simulink model "deep_sim_0"  (R2025b)
settings: Solver=FixedStepAuto  StartTime=0.0  StopTime=300  FixedStep=.01  RelTol=1e-3
undefined symbols (not defined in the file or in its folder): battery_builder_rtmsupport, gcbh
libraries: Batteries_lib x15, nesl_utility x5, fl_lib x4, ee_lib x1
(part 2 of 2)

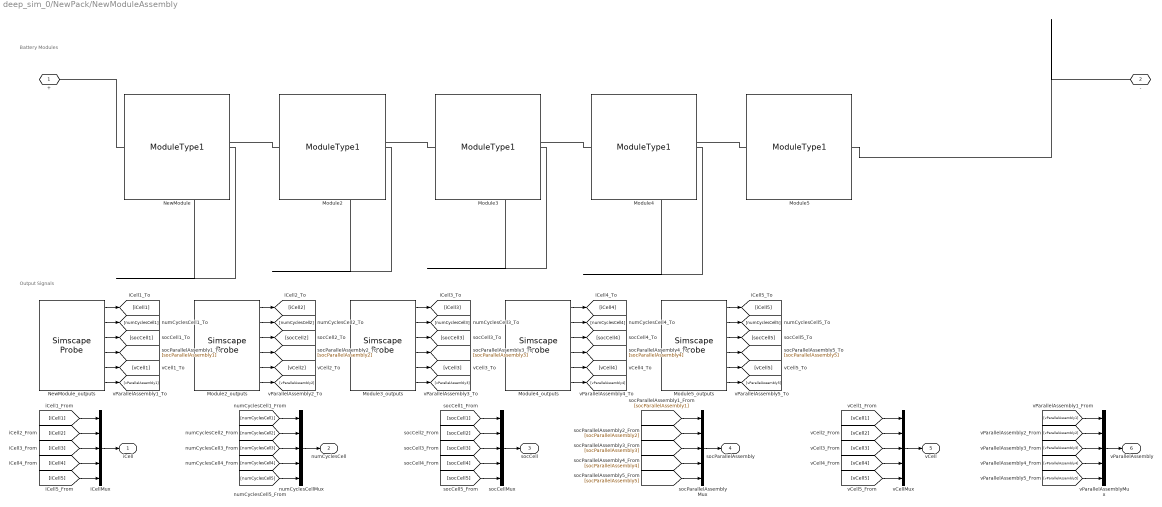
== system deep_sim_0/NewPack/NewModuleAssembly ==
  note: Battery Modules
  note: Output Signals
  Module{2..5} (4 alike) : Batteries_lib/Modules/ModuleType1  SOC_vecCell=[0, .01, .02, .03, .04, .05, .06, .07, .08, .09, .1, .11, .12, .13, .14, .15, .16, .17, .18, .19, .2, .21, .22, .23, .24, .25, .26, .27, .28, .29, .3, .31, .32, .33, .34, .35, .36, .37, .38, .39, .4, .41, .42, .43, .44, .45, .46, .47, .48, .49, .5, .51, .52, .53, .54, .55, .56, .57, .58, .59, .6, .61, .62, .63, .64, .65, .66, .67, .68, .69, .7, .71, .72, .73, .74, .75, .76, .77, .78, .79, .8, .81, .82, .83, .84, .85, .86, .87, .88, .89, .9, .91, .92, .93, .94, .95, .96, .97, .98, .99, 1]  V0_vecCell=[3.17242, 3.18272, 3.19302, 3.20331, 3.21361, 3.22391, 3.23421, 3.24451, 3.25481, 3.2651, 3.2754, 3.2857, 3.296, 3.3063, 3.31659, 3.32689, 3.33719, 3.34749, 3.35779, 3.36809, 3.37838, 3.38868, 3.39898, 3.40928, 3.41958, 3.42988, 3.44017, 3.45047, 3.46077, 3.47107, 3.48137, 3.49166, 3.50196, 3.51226, 3.52256, 3.53286, 3.54316, 3.55345, 3.56375, 3.57405, 3.58435, 3.59465, 3.60495, 3.61524, 3.62554, 3.63584, 3.64614, 3.65644, 3.66673, 3.67703, 3.68733, 3.69763, 3.71041, 3.72113, 3.72997, 3.73882, 3.74912, 3.75936, 3.76951, 3.7791, 3.78865, 3.79787, 3.80709, 3.8161, 3.82509, 3.83409, 3.84308, 3.85207, 3.86107, 3.87006, 3.87901, 3.88831, 3.89824, 3.90887, 3.91951, 3.93012, 3.94073, 3.95138, 3.96184, 3.97226, 3.98268, 3.99311, 4.0032, 4.01221, 4.01944, 4.02668, 4.03286, 4.03874, 4.04383, 4.0488, 4.05377, 4.05873, 4.06312, 4.06753, 4.07333, 4.08117, 4.08904, 4.09911, 4.11111, 4.13802, 4.16831] V  V_rangeCell=[2.25, Inf] V  R0_vecCell=[.02095, .01921, .01774, .0166, .01557, .01469, .01398, .01338, .01283, .01239, .01196, .01155, .01116, .01079, .01042, .01007, .00974, .00949, .00924, .009, .00876, .00855, .00843, .00832, .00826, .00825, .00825, .00826, .00827, .00828, .0083, .00834, .00838, .00842, .00848, .00855, .00863, .00871, .00879, .00887, .00895, .00903, .00911, .00918, .00925, .00931, .00938, .00946, .00953, .00961, .00968, .00976, .00991, .01, .01003, .01006, .01013, .01022, .0103, .01037, .01043, .01049, .01055, .01061, .01066, .01072, .01077, .01082, .01088, .01093, .01099, .01105, .01114, .01125, .01136, .01148, .01161, .01175, .01188, .01202, .01215, .01228, .01241, .01253, .01261, .01269, .01275, .0128, .01285, .01289, .01294, .01298, .01296, .01292, .01292, .01288, .01282, .0128, .01232, .01214, .00952] Ohm  AHCell=4.493 A*hr  extrapolation_optionCell=simscape.enum.extrapolation.nearest  P=1  S=13  iCell_specify=off  iCell_priority=None  iCell=0 A  iCell_nominal_specify=off  iCell_nominal_value=1  iCell_nominal_unit=A  vCell_specify=off  vCell_priority=None  vCell=0 V  vCell_nominal_specify=off  vCell_nominal_value=1  vCell_nominal_unit=V  socCell_specify=on  socCell_priority=High  socCell=0.08  socCell_nominal_specify=off  socCell_nominal_value=1  socCell_nominal_unit=1  numCyclesCell_specify=off  numCyclesCell_priority=High  numCyclesCell=0  numCyclesCell_nominal_specify=off  numCyclesCell_nominal_value=1  numCyclesCell_nominal_unit=1  vParallelAssembly_specify=off  vParallelAssembly_priority=None  vParallelAssembly=repmat(0, 13, 1) V  vParallelAssembly_nominal_specify=off  vParallelAssembly_nominal_value=1  vParallelAssembly_nominal_unit=V  socParallelAssembly_specify=off  socParallelAssembly_priority=None  socParallelAssembly=repmat(1, 13, 1)  socParallelAssembly_nominal_specify=off  socParallelAssembly_nominal_value=1  socParallelAssembly_nominal_unit=1
      settings: InternalSimscapePortConfiguration="{\"Bottom\":[{\"id\":\"n\",\"label\":\"-\",\"type\":\"foundation.electrical.electrical\"}],\"Left\":[],\"Right\":[],\"Top\":[{\"id\":\"p\",\"label\":\"+\",\"type\":\"foundation.electrical.electrical\"}]}"
  Module2_outputs : SimscapeProbe  BoundBlock=227  Variables="{\"iCell\":{\"Probing\":\"ON\"},\"numCyclesCell\":{\"Probing\":\"ON\"},\"socCell\":{\"Probing\":\"ON\"},\"socParallelAssembly\":{\"Probing\":\"ON\"},\"vCell\":{\"Probing\":\"ON\"},\"vParallelAssembly\":{\"Probing\":\"ON\"}}"
  Module3_outputs : SimscapeProbe  BoundBlock=229  Variables="{\"iCell\":{\"Probing\":\"ON\"},\"numCyclesCell\":{\"Probing\":\"ON\"},\"socCell\":{\"Probing\":\"ON\"},\"socParallelAssembly\":{\"Probing\":\"ON\"},\"vCell\":{\"Probing\":\"ON\"},\"vParallelAssembly\":{\"Probing\":\"ON\"}}"
  Module4_outputs : SimscapeProbe  BoundBlock=231  Variables="{\"iCell\":{\"Probing\":\"ON\"},\"numCyclesCell\":{\"Probing\":\"ON\"},\"socCell\":{\"Probing\":\"ON\"},\"socParallelAssembly\":{\"Probing\":\"ON\"},\"vCell\":{\"Probing\":\"ON\"},\"vParallelAssembly\":{\"Probing\":\"ON\"}}"
  Module5_outputs : SimscapeProbe  BoundBlock=233  Variables="{\"iCell\":{\"Probing\":\"ON\"},\"numCyclesCell\":{\"Probing\":\"ON\"},\"socCell\":{\"Probing\":\"ON\"},\"socParallelAssembly\":{\"Probing\":\"ON\"},\"vCell\":{\"Probing\":\"ON\"},\"vParallelAssembly\":{\"Probing\":\"ON\"}}"
  NewModule : Batteries_lib/Modules/ModuleType1  SOC_vecCell=[0, .01, .02, .03, .04, .05, .06, .07, .08, .09, .1, .11, .12, .13, .14, .15, .16, .17, .18, .19, .2, .21, .22, .23, .24, .25, .26, .27, .28, .29, .3, .31, .32, .33, .34, .35, .36, .37, .38, .39, .4, .41, .42, .43, .44, .45, .46, .47, .48, .49, .5, .51, .52, .53, .54, .55, .56, .57, .58, .59, .6, .61, .62, .63, .64, .65, .66, .67, .68, .69, .7, .71, .72, .73, .74, .75, .76, .77, .78, .79, .8, .81, .82, .83, .84, .85, .86, .87, .88, .89, .9, .91, .92, .93, .94, .95, .96, .97, .98, .99, 1]  V0_vecCell=[3.17242, 3.18272, 3.19302, 3.20331, 3.21361, 3.22391, 3.23421, 3.24451, 3.25481, 3.2651, 3.2754, 3.2857, 3.296, 3.3063, 3.31659, 3.32689, 3.33719, 3.34749, 3.35779, 3.36809, 3.37838, 3.38868, 3.39898, 3.40928, 3.41958, 3.42988, 3.44017, 3.45047, 3.46077, 3.47107, 3.48137, 3.49166, 3.50196, 3.51226, 3.52256, 3.53286, 3.54316, 3.55345, 3.56375, 3.57405, 3.58435, 3.59465, 3.60495, 3.61524, 3.62554, 3.63584, 3.64614, 3.65644, 3.66673, 3.67703, 3.68733, 3.69763, 3.71041, 3.72113, 3.72997, 3.73882, 3.74912, 3.75936, 3.76951, 3.7791, 3.78865, 3.79787, 3.80709, 3.8161, 3.82509, 3.83409, 3.84308, 3.85207, 3.86107, 3.87006, 3.87901, 3.88831, 3.89824, 3.90887, 3.91951, 3.93012, 3.94073, 3.95138, 3.96184, 3.97226, 3.98268, 3.99311, 4.0032, 4.01221, 4.01944, 4.02668, 4.03286, 4.03874, 4.04383, 4.0488, 4.05377, 4.05873, 4.06312, 4.06753, 4.07333, 4.08117, 4.08904, 4.09911, 4.11111, 4.13802, 4.16831] V  V_rangeCell=[2.25, Inf] V  R0_vecCell=[.02095, .01921, .01774, .0166, .01557, .01469, .01398, .01338, .01283, .01239, .01196, .01155, .01116, .01079, .01042, .01007, .00974, .00949, .00924, .009, .00876, .00855, .00843, .00832, .00826, .00825, .00825, .00826, .00827, .00828, .0083, .00834, .00838, .00842, .00848, .00855, .00863, .00871, .00879, .00887, .00895, .00903, .00911, .00918, .00925, .00931, .00938, .00946, .00953, .00961, .00968, .00976, .00991, .01, .01003, .01006, .01013, .01022, .0103, .01037, .01043, .01049, .01055, .01061, .01066, .01072, .01077, .01082, .01088, .01093, .01099, .01105, .01114, .01125, .01136, .01148, .01161, .01175, .01188, .01202, .01215, .01228, .01241, .01253, .01261, .01269, .01275, .0128, .01285, .01289, .01294, .01298, .01296, .01292, .01292, .01288, .01282, .0128, .01232, .01214, .00952] Ohm  AHCell=4.493 A*hr  extrapolation_optionCell=simscape.enum.extrapolation.nearest  P=1  S=13  iCell_specify=off  iCell_priority=None  iCell=0 A  iCell_nominal_specify=off  iCell_nominal_value=1  iCell_nominal_unit=A  vCell_specify=off  vCell_priority=None  vCell=0 V  vCell_nominal_specify=off  vCell_nominal_value=1  vCell_nominal_unit=V  socCell_specify=on  socCell_priority=High  socCell=0.08  socCell_nominal_specify=off  socCell_nominal_value=1  socCell_nominal_unit=1  numCyclesCell_specify=off  numCyclesCell_priority=High  numCyclesCell=0  numCyclesCell_nominal_specify=off  numCyclesCell_nominal_value=1  numCyclesCell_nominal_unit=1  vParallelAssembly_specify=off  vParallelAssembly_priority=None  vParallelAssembly=repmat(0, 13, 1) V  vParallelAssembly_nominal_specify=off  vParallelAssembly_nominal_value=1  vParallelAssembly_nominal_unit=V  socParallelAssembly_specify=off  socParallelAssembly_priority=None  socParallelAssembly=repmat(1, 13, 1)  socParallelAssembly_nominal_specify=off  socParallelAssembly_nominal_value=1  socParallelAssembly_nominal_unit=1
      settings: InternalSimscapePortConfiguration="{\"Bottom\":[{\"id\":\"n\",\"label\":\"-\",\"type\":\"foundation.electrical.electrical\"}],\"Left\":[],\"Right\":[],\"Top\":[{\"id\":\"p\",\"label\":\"+\",\"type\":\"foundation.electrical.electrical\"}]}"
  NewModule_outputs : SimscapeProbe  BoundBlock=235  Variables="{\"iCell\":{\"Probing\":\"ON\"},\"numCyclesCell\":{\"Probing\":\"ON\"},\"socCell\":{\"Probing\":\"ON\"},\"socParallelAssembly\":{\"Probing\":\"ON\"},\"vCell\":{\"Probing\":\"ON\"},\"vParallelAssembly\":{\"Probing\":\"ON\"}}"
  iCellMux : Mux  Inputs=5
  numCyclesCellMux : Mux  Inputs=5
  socCellMux : Mux  Inputs=5
  socParallelAssemblyMux : Mux  Inputs=5
  vCellMux : Mux  Inputs=5
  vParallelAssemblyMux : Mux  Inputs=5
  + : PMIOPort  Side=Left
  - : PMIOPort  Port=2  Side=Right
  iCell : Outport
  numCyclesCell : Outport  Port=2
  socCell : Outport  Port=3
  socParallelAssembly : Outport  Port=4
  vCell : Outport  Port=5
  vParallelAssembly : Outport  Port=6
  wires:
  NewModule_outputs/1 -> [iCell1]
  iCellMux/1 -> iCell/1
  [iCell1] -> iCellMux/1
  NewModule_outputs/2 -> [numCyclesCell1]
  numCyclesCellMux/1 -> numCyclesCell/1
  [numCyclesCell1] -> numCyclesCellMux/1
  NewModule_outputs/3 -> [socCell1]
  socCellMux/1 -> socCell/1
  [socCell1] -> socCellMux/1
  NewModule_outputs/4 -> [socParallelAssembly1]
  socParallelAssemblyMux/1 -> socParallelAssembly/1
  [socParallelAssembly1] -> socParallelAssemblyMux/1
  NewModule_outputs/5 -> [vCell1]
  vCellMux/1 -> vCell/1
  [vCell1] -> vCellMux/1
  NewModule_outputs/6 -> [vParallelAssembly1]
  vParallelAssemblyMux/1 -> vParallelAssembly/1
  [vParallelAssembly1] -> vParallelAssemblyMux/1
  Module2_outputs/1 -> [iCell2]
  [iCell2] -> iCellMux/2
  Module2_outputs/2 -> [numCyclesCell2]
  [numCyclesCell2] -> numCyclesCellMux/2
  Module2_outputs/3 -> [socCell2]
  [socCell2] -> socCellMux/2
  Module2_outputs/4 -> [socParallelAssembly2]
  [socParallelAssembly2] -> socParallelAssemblyMux/2
  Module2_outputs/5 -> [vCell2]
  [vCell2] -> vCellMux/2
  Module2_outputs/6 -> [vParallelAssembly2]
  [vParallelAssembly2] -> vParallelAssemblyMux/2
  Module3_outputs/1 -> [iCell3]
  [iCell3] -> iCellMux/3
  Module3_outputs/2 -> [numCyclesCell3]
  [numCyclesCell3] -> numCyclesCellMux/3
  Module3_outputs/3 -> [socCell3]
  [socCell3] -> socCellMux/3
  Module3_outputs/4 -> [socParallelAssembly3]
  [socParallelAssembly3] -> socParallelAssemblyMux/3
  Module3_outputs/5 -> [vCell3]
  [vCell3] -> vCellMux/3
  Module3_outputs/6 -> [vParallelAssembly3]
  [vParallelAssembly3] -> vParallelAssemblyMux/3
  Module4_outputs/1 -> [iCell4]
  [iCell4] -> iCellMux/4
  Module4_outputs/2 -> [numCyclesCell4]
  [numCyclesCell4] -> numCyclesCellMux/4
  Module4_outputs/3 -> [socCell4]
  [socCell4] -> socCellMux/4
  Module4_outputs/4 -> [socParallelAssembly4]
  [socParallelAssembly4] -> socParallelAssemblyMux/4
  Module4_outputs/5 -> [vCell4]
  [vCell4] -> vCellMux/4
  Module4_outputs/6 -> [vParallelAssembly4]
  [vParallelAssembly4] -> vParallelAssemblyMux/4
  Module5_outputs/1 -> [iCell5]
  [iCell5] -> iCellMux/5
  Module5_outputs/2 -> [numCyclesCell5]
  [numCyclesCell5] -> numCyclesCellMux/5
  Module5_outputs/3 -> [socCell5]
  [socCell5] -> socCellMux/5
  Module5_outputs/4 -> [socParallelAssembly5]
  [socParallelAssembly5] -> socParallelAssemblyMux/5
  Module5_outputs/5 -> [vCell5]
  [vCell5] -> vCellMux/5
  Module5_outputs/6 -> [vParallelAssembly5]
  [vParallelAssembly5] -> vParallelAssemblyMux/5
  connections:
  Module2/LConn1 -- NewModule/RConn1
  Module3/LConn1 -- Module2/RConn1
  Module4/LConn1 -- Module3/RConn1
  Module5/LConn1 -- Module4/RConn1
  NewModule/LConn1 -- +/RConn1
  Module5/RConn1 -- -/RConn1

== matlab function deep_sim_0/Charger/Charger_core ==
  settings: updateMethod=DISCRETE  sampleTime=0.01
  data: pack_meas input; I_chg_cmd output; enable input; I_limit input; P_chg_cmd output; mode output; V_set output; I_set output; done output
function [I_chg_cmd, P_chg_cmd, mode, V_set, I_set, done] = ...
        fcn(pack_meas, enable, I_limit)
%#codegen
%CHARGER_CORE  Generated by bcp.ChargerBuilder. Do not edit here.
%
%  Edit bcp.ChargerConfig (or the Charger tab of bcpApp) and re-insert the
%  block. Changes made in this window are overwritten by the next insert.
%
%  pack_meas indices are fixed by bcp.Signals:
%    1 V_pack  2 V_cell_min  3 V_cell_max  4 SOC_pack  5 SOC_min
%    6 SOC_max 7 I_pack (charge-positive)

%% ===== WHAT THIS SUPPLY CAN SOURCE =================================
%%  These two are HARDWARE ratings, not the charge rate. The charge rate
%%  arrives on the I_limit input from the BMS block, and this block
%%  commands the lower of the two -- so to charge faster you change one
%%  number in the BMS (I_CHG_MAX_A), not anything here.
%%
%%  Change these only when you are modelling a different power supply.
%%  Setting either below the BMS limit makes this block the thing that
%%  limits the charge, which is legitimate but is worth knowing you did:
%%  bcp.Project.check() says so before you run.
I_SUPPLY_MAX_A = 13.5;
P_SUPPLY_MAX_W = 11056.5;
%% ===================================================================

P = struct( ...
        'Ts', 0.01, ...
        'SeriesCount', 195, ...
        'I_cc_A', 13.5, ...
        'I_taper_A', 0.22465, ...
        'I_precharge_A', 0.4493, ...
        'V_cv_cell', 4.2, ...
        'V_cv_pack', 819, ...
        'V_precharge_cell', 3, ...
        'V_recharge_cell', 4.05, ...
        'Kp_cell', 30.9917355372, ...
        'Ki_cell', 61.9834710744, ...
        'Kp_pack', 0.158931977114, ...
        'Ki_pack', 0.317863954228, ...
        't_term_s', 2, ...
        'V_term_band', 0.03, ...
        'Mode_Hyst_frac', 0.03, ...
        't_mode_min_s', 0.25, ...
        'ForceMode', 0);
P.I_cc_A = I_SUPPLY_MAX_A;

%  The CV loop is handed the HIGHEST cell, not the pack average. On a pack
%  with real cell spread those are different constraints, and the per-cell
%  one is what keeps a cell out of over-voltage. See bcp_charger.
[I_chg_cmd, P_chg_cmd, mode, V_set, I_set, done] = bcp_charger( ...
    pack_meas(1), pack_meas(3), pack_meas(7), enable, I_limit, P);

%  Supply power ceiling, applied last so it cannot be reasoned around by the
%  control law: a real supply simply cannot deliver more than this.
if P_chg_cmd > P_SUPPLY_MAX_W
    P_chg_cmd = P_SUPPLY_MAX_W;
    if pack_meas(1) > 1
        I_chg_cmd = P_chg_cmd / pack_meas(1);
    end
end
end

== matlab function deep_sim_0/BMS/BMS_core ==
  settings: updateMethod=DISCRETE  sampleTime=0.01
  data: t input; P_load_cmd output; Vcell input; SOCcell input; Icell input; Tmax input; P_chg input; chg_done input; reset input; P_net_cmd output; chg_enable output; I_chg_limit output; pack_meas output; contactor output; state output; faults output; diag output
function [P_load_cmd, P_net_cmd, chg_enable, I_chg_limit, pack_meas, ...
          contactor, state, faults, diag] = ...
        fcn(t, Vcell, SOCcell, Icell, Tmax, P_chg, chg_done, reset)
%#codegen
%BMS_CORE  Generated by bcp.BmsBuilder. Do not edit here.
%
%  Edit bcp.BmsConfig / bcp.LoadSignal (or the Load and BMS tabs of bcpApp)
%  and re-insert the block. Changes made in this window are overwritten by
%  the next insert, and are invisible to the tests.
%
%  Sign convention inside this function: POSITIVE CURRENT = CHARGING.
%  Load power is DRAW-POSITIVE. The two meet at P_net_cmd.

%% ===== THE CHARGE-RATE KNOB =========================================
%%  ONE number sets how fast this system charges. It leaves this block on
%%  I_chg_limit, and the charger commands the lower of it and its own
%%  supply rating -- so nothing in the charger block has to match it,
%%  and the two cannot disagree.
%%
%%  Raising it does NOT bypass protection. Both charge over-current trips
%%  are computed from it a few lines down, so they move with the operating
%%  point instead of becoming a ceiling you forgot to raise.
%%
%%  Editing it here is a fine quick experiment. The next insert overwrites
%%  it, so put the value you settle on into bcp.BmsConfig.I_chg_max_A --
%%  or the Charge current field in the UI, which is the same thing.
I_CHG_MAX_A = 4.35;    %% amps at the pack terminals
OC_TRIP_X   = 1.25011494253;    %% sustained charge trip / I_CHG_MAX_A, confirmed over 10 s
OC_PEAK_X   = 1.6;    %% fast charge trip / I_CHG_MAX_A, confirmed over 0.1 s
%% ====================================================================

MON = struct( ...
        'SeriesCount', 195, ...
        'I_sign', 1, ...
        'SOC_in_percent', false, ...
        'SOC_clamp', true);
PRO = struct( ...
        'Ts', 0.01, ...
        'V_ov_trip', 4.25, ...
        'V_ov_clear', 4.15, ...
        'V_uv_trip', 2.5, ...
        'V_uv_clear', 3, ...
        't_v_trip', 0.5, ...
        'I_chg_trip', 5.438, ...
        'I_chg_peak', 6.96, ...
        'I_dch_trip', 49.5, ...
        'I_dch_peak', 74.3, ...
        't_i_trip', 0.1, ...
        't_i_cont', 10, ...
        'T_ot_trip', 60, ...
        'T_ot_clear', 50, ...
        'T_ut_trip', 0, ...
        't_T_trip', 5, ...
        'AutoRecover', true, ...
        't_recover', 2, ...
        'Q_uv_reset_Ah', 0.0225, ...
        'Retry_Backoff_x', 3, ...
        't_recover_max_s', 60, ...
        't_retry_window_s', 30, ...
        'N_retry_max', 3);
ARB = struct( ...
        'Ts', 0.01, ...
        'ChargeEnabled', true, ...
        'AllowConcurrent', false, ...
        't_quiet_s', 1, ...
        'SOC_stop', 0.95, ...
        'SOC_restart', 0.85, ...
        'V_recharge', 4.05, ...
        'I_chg_max_A', 4.35, ...
        'I_chg_headroom_A', 5);
LIM = struct( ...
        'Ts', 0.01, ...
        'Enabled', false, ...
        'V_fold_end', 2.58, ...
        'V_fold_start', 2.78, ...
        'I_fold_start', 66.87, ...
        'I_fold_end', 74.3, ...
        'Fold_Fall_per_s', 20, ...
        'Fold_Rise_per_s', 0.25, ...
        'Fold_Floor', 0, ...
        'I_learn_A', 6.687, ...
        't_softstart_s', 0.5);
LOAD = struct( ...
        'Ts', 0.01, ...
        'Waveform', 3, ...
        'StartTime_s', 5, ...
        'StopTime_s', Inf, ...
        'Offset_W', 0, ...
        'Amplitude_W', 31250, ...
        'Frequency_Hz', 0.05, ...
        'Phase_deg', 0, ...
        'Duty_pct', 10, ...
        'Pmin_W', 0, ...
        'Pmax_W', 35000, ...
        'Slew_W_per_s', 625000, ...
        'IdleThreshold_W', 5);
OUT_SIGN = 1;

%  The knob, applied. These three lines are the whole reason the charge
%  rate is one number: every threshold and every limit below reads them.
PRO.I_chg_trip  = I_CHG_MAX_A * OC_TRIP_X;
PRO.I_chg_peak  = I_CHG_MAX_A * OC_PEAK_X;
ARB.I_chg_max_A = I_CHG_MAX_A;

%  Reduce the temperature input to a scalar. With the temperature port off
%  this is a constant and the reduction costs nothing; with it on, whatever
%  your battery model exports becomes the hottest reading, which is what
%  protection wants. It also pins the diag output at exactly 10 elements: a
%  vector arriving here would widen the fault flags and the port with them,
%  and that compile error lands nowhere near the wire that caused it.
T_hot = max(Tmax(:));

%  1. Reduce the per-cell arrays to pack scalars. soc_raw is the UNCLAMPED
%     [min; max] SOC the battery model reported -- kept for diag(17), because
%     a Simscape table_battery integrates coulombs with no floor and will
%     report a negative SOC forever once the pack is past empty.
[pack_meas, soc_raw] = bcp_pack_monitor(Vcell, SOCcell, Icell, MON);

%  2. What does the load waveform ask for at this instant?
[P_demand, demandPresent] = bcp_load_scheduler(t, LOAD);

%  3. Protection, on the pack extremes.
[contactor, chg_ok, dch_ok, state, faults, flags, pinfo] = bcp_protection( ...
    pack_meas(2), pack_meas(3), T_hot, pack_meas(7), reset > 0.5, PRO);

%  4. The load, limited. A discharge inhibit has to inhibit the discharge --
%     the load is the only discharge path in this model -- but a BINARY
%     inhibit on a constant-power load oscillates, because cutting the load
%     removes the sag that tripped it. bcp_load_limiter puts a continuous
%     limit in front of the trip, the way a production BMS publishes a
%     discharge limit the inverter must obey, so protection stays a backstop.
%     alg/bcp_load_limiter.m derives the oscillation and the fix in full.
%
%     The GATED, LIMITED value is what counts as "the load is active", and
%     the order matters. Feeding the ungated demand to the arbiter would mean
%     an under-voltage fault holds the load flag high, the arbiter sees a busy
%     load and refuses to charge, and the pack sits at its floor forever --
%     deadlocked by its own protection, with a charger idle beside it. The
%     cure for under-voltage is a charge.
[P_load, dclFrac, limState] = bcp_load_limiter( ...
    P_demand, pack_meas(2), pack_meas(7), dch_ok, LIM);
loadActive = double(abs(P_load) > LOAD.IdleThreshold_W);

%  5. Arbitrate. The load has already happened; this decides what is left.
[chg_enable, I_chg_limit, reason] = bcp_arbiter( ...
    loadActive, pack_meas(4), pack_meas(3), chg_ok, chg_done, ARB);

%  6. Shape the outputs.
P_load_cmd = OUT_SIGN * P_load;
P_net_cmd  = OUT_SIGN * (P_load - P_chg);

%  Preallocated, so diag is 17 wide at compile time whatever code generation
%  infers about the pieces going into it. Channel names: bcp.Signals.diagNames.
diag = zeros(17,1);
diag(1) = demandPresent;
diag(2) = loadActive;
diag(3) = reason;
diag(4) = dch_ok;
diag(5:10) = flags(1:6);
diag(11) = dclFrac;         % 0..1, the fraction of demand allowed through
diag(12) = limState;        % which limit is binding, bcp.Signals.limitState
diag(13) = pinfo(1);        % automatic recoveries inside the retry window
diag(14) = pinfo(2);        % 1 = auto-recovery withdrawn, reset only
diag(15) = pinfo(3);        % Ah charged since the under-voltage latch
diag(16) = pinfo(4);        % clear-band dwell recovery currently requires
diag(17) = soc_raw(1);      % UNCLAMPED min SOC -- negative means past empty
end
